simulink model "One_Shot_Simulation"  (R2018b)
settings: Solver=VariableStepAuto  StartTime=0.0  StopTime=5  RelTol=1e-3
libraries: truetime x1
settings Model: Creator=ortegafausto  LastModifiedBy=of
settings SFSimCC: SimUseLocalCustomCode=off
settings RTWCC: RTWUseLocalCustomCode=off
settings CodeAppCC: StateflowObjectComments=on
settings SimscapeCC: SimscapeNormalizeSystem=off

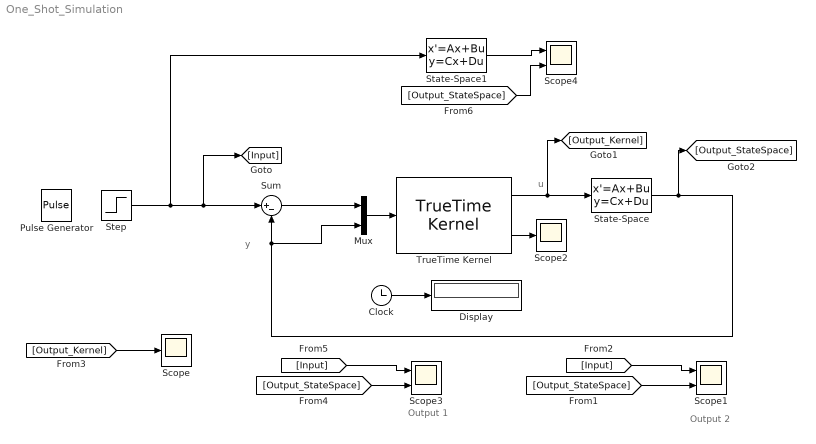
== system One_Shot_Simulation ==
  note: Output 2
  note: Output 1
  note: y
  note: u
  Clock : Clock
  Display : Display
  Mux : Mux  Inputs=2
  Pulse Generator : DiscretePulseGenerator  PulseType=Time based  Amplitude=2.4  Period=1  PulseWidth=50
  Scope : Scope
  Scope1 : Scope  NumInputPorts=2
  Scope2 : Scope
  Scope3 : Scope  NumInputPorts=2
  Scope4 : Scope  NumInputPorts=2
  State-Space : StateSpace  A=[0 1; -918.27 -90.90]  B=[0; 918.27]  C=[1 0]  D=0  InitialCondition=0
  State-Space1 : StateSpace  A=[0 1; -918.27 -90.90]  B=[0; 918.27]  C=[1 0]  D=0  InitialCondition=0
  Step : Step  After=2.4  SampleTime=0
  Sum : Sum  Inputs=|+-
  TrueTime Kernel : truetime/TrueTime Kernel  sfun=one_shot_init  args=[]  ninputsoutputs=[2 1]  ntriggers=0  trigtype=falling  nwnodenbr=[]  clockoffsetdrift=[0 0]  schedoutput=on  battery=off  poweroutput=off
  wires:
  Clock/1 -> Display/1
  TrueTime Kernel/2 -> Scope2/1
  State-Space/1 -> [Output_StateSpace], Sum/2, Mux/2
  Mux/1 -> TrueTime Kernel/1
  Sum/1 -> Mux/1
  TrueTime Kernel/1 -> [Output_Kernel], State-Space/1
  [Output_StateSpace] -> Scope1/2
  [Input] -> Scope1/1
  [Input] -> Scope3/1
  [Output_StateSpace] -> Scope3/2
  [Output_Kernel] -> Scope/1
  Step/1 -> State-Space1/1, [Input], Sum/1
  State-Space1/1 -> Scope4/1
  [Output_StateSpace] -> Scope4/2
